simulink model "real_motor_awp"  (R2025b)
settings: Solver=VariableStepAuto  StartTime=0.0  StopTime=3  RelTol=1e-3
undefined symbols (not defined in the file): C, F, fc, G, K, K_awp, K_I, L, T, x_r
libraries: simulink x2
settings Model: Creator=noeliarosales  LastModifiedBy=noeliarosales

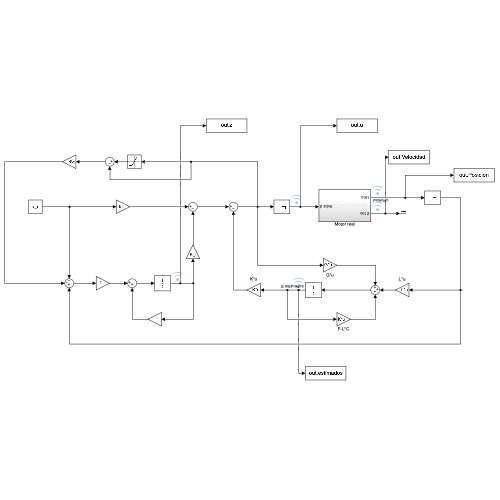
[thumbnail: Simulink's stored preview of the top-level diagram]
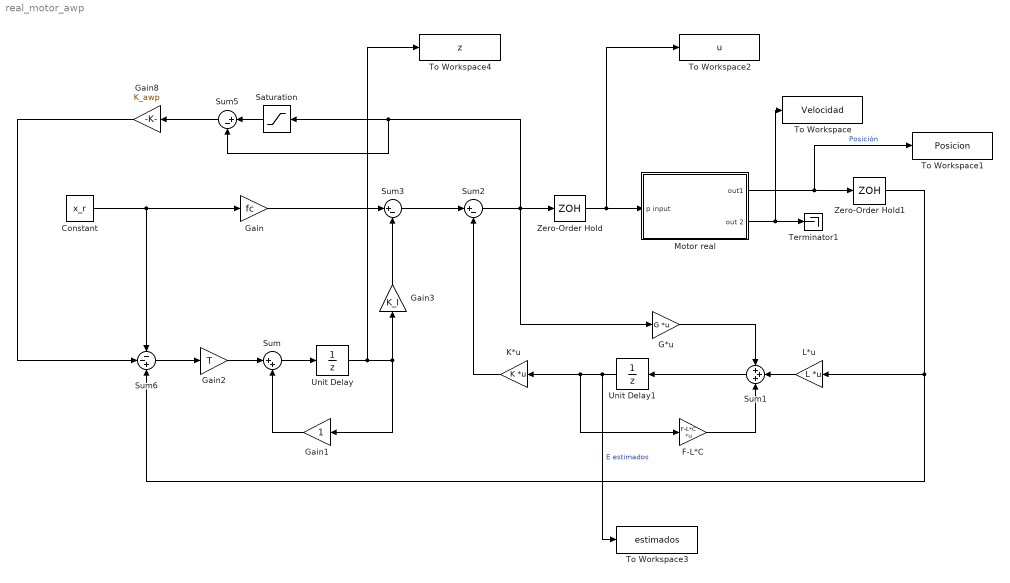
== system real_motor_awp ==
  Constant : Constant  Value=x_r
  F-L*C : Gain  Gain=F-L*C  Multiplication=Matrix(K*u)
  G*u : Gain  Gain=G  Multiplication=Matrix(K*u)
  Gain : Gain  Gain=fc
  Gain1 : Gain
  Gain2 : Gain  Gain=T
  Gain3 : Gain  Gain=K_I
  Gain8 : Gain  Gain=K_awp
  K*u : Gain  Gain=K  Multiplication=Matrix(K*u)
  L*u : Gain  Gain=L  Multiplication=Matrix(K*u)
  Motor real : Subsystem
  Saturation : Saturate  UpperLimit=100/12
  Sum : Sum  Inputs=|++
  Sum1 : Sum  Inputs=+++
  Sum2 : Sum  Inputs=|+-
  Sum3 : Sum  Inputs=|+-
  Sum5 : Sum  Inputs=|+-
  Sum6 : Sum  Inputs=--+
  Terminator1 : Terminator
  To Workspace : ToWorkspace  VariableName=Velocidad  SaveFormat=Timeseries  SampleTime=-1
  To Workspace1 : ToWorkspace  VariableName=Posicion  SaveFormat=Timeseries  SampleTime=-1
  To Workspace2 : ToWorkspace  VariableName=u  SaveFormat=Timeseries  SampleTime=-1
  To Workspace3 : ToWorkspace  VariableName=estimados  SaveFormat=Timeseries  SampleTime=-1
  To Workspace4 : ToWorkspace  VariableName=z  SaveFormat=Timeseries  SampleTime=-1
  Unit Delay : UnitDelay  SampleTime=-1  HasFrameUpgradeWarning=on
  Unit Delay1 : UnitDelay  SampleTime=-1  HasFrameUpgradeWarning=on
  Zero-Order Hold : ZeroOrderHold  SampleTime=T
  Zero-Order Hold1 : ZeroOrderHold  SampleTime=T
  wires:
  Zero-Order Hold/1 -> To Workspace2/1, Motor real/1(p input)
  Zero-Order Hold1/1 -> Sum6/3, L*u/1
  L*u/1 -> Sum1/2
  G*u/1 -> Sum1/1
  Sum1/1 -> Unit Delay1/1
  Constant/1 -> Sum6/1, Gain/1
  Gain3/1 -> Sum3/2
  F-L*C/1 -> Sum1/3
  Sum6/1 -> Gain2/1
  Sum3/1 -> Sum2/1
  Unit Delay1/1 -> To Workspace3/1, K*u/1, F-L*C/1  "E estimados"
  Sum/1 -> Unit Delay/1
  Motor real/1(out1) -> To Workspace1/1, Zero-Order Hold1/1  "Posición"
  Gain/1 -> Sum3/1
  K*u/1 -> Sum2/2
  Gain1/1 -> Sum/2
  Sum2/1 -> Sum5/2, Saturation/1, G*u/1, Zero-Order Hold/1
  Motor real/2(out 2) -> To Workspace/1, Terminator1/1
  Gain2/1 -> Sum/1
  Unit Delay/1 -> To Workspace4/1, Gain3/1, Gain1/1
  Sum5/1 -> Gain8/1
  Saturation/1 -> Sum5/1
  Gain8/1 -> Sum6/2

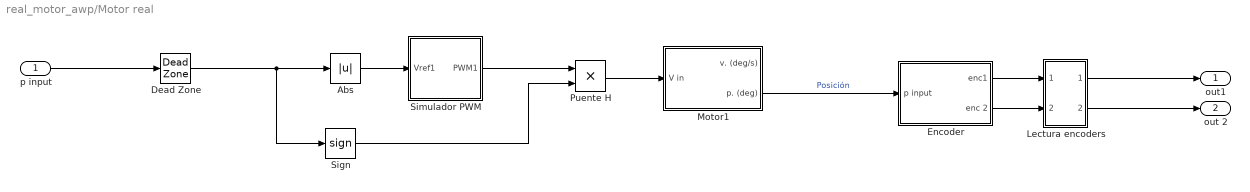
== system real_motor_awp/Motor real ==
  p input : Inport
  " Encoder" : Subsystem
  Abs : Abs  SaturateOnIntegerOverflow=off
  Dead Zone : DeadZone
  Lectura encoders : Subsystem
  Motor1 : Subsystem
  Puente H : Product
  Sign : Signum
  Simulador PWM : Subsystem
  out1 : Outport
  out 2 : Outport  Port=2
  wires:
  Lectura encoders/2(Encoder B) -> out 2/1
  Sign/1 -> Puente H/2
  Abs/1 -> Simulador PWM/1(Vref1)
  " Encoder"/1(enc1) -> Lectura encoders/1(enc1)
  " Encoder"/2(enc 2) -> Lectura encoders/2(enc 2)
  Puente H/1 -> Motor1/1(V in)
  Dead Zone/1 -> Sign/1, Abs/1
  Lectura encoders/1(Encoder A) -> out1/1
  Motor1/2(p. (deg)) -> " Encoder"/1(p input)  "Posición"
  Simulador PWM/1(PWM1) -> Puente H/1
  p input/1 -> Dead Zone/1

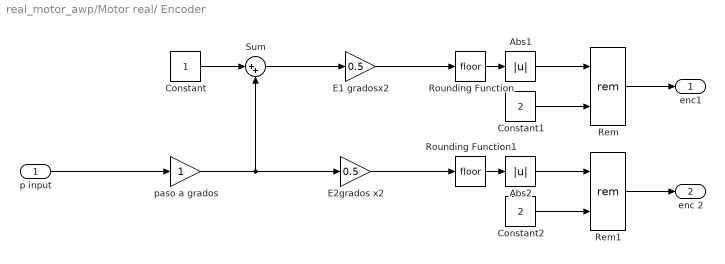
== system real_motor_awp/Motor real/ Encoder ==
  p input : Inport
  Abs1 : Abs  SaturateOnIntegerOverflow=off
  Abs2 : Abs  SaturateOnIntegerOverflow=off
  Constant : Constant
  Constant1 : Constant  Value=2
  Constant2 : Constant  Value=2
  E1 gradosx2 : Gain  Gain=0.5
  E2grados x2 : Gain  Gain=0.5
  Rem : Math  Operator=rem
  Rem1 : Math  Operator=rem
  Rounding Function : Rounding
  Rounding Function1 : Rounding
  Sum : Sum  Inputs=|++
  paso a grados : Gain
  enc1 : Outport
  enc 2 : Outport  Port=2
  wires:
  paso a grados/1 -> E2grados x2/1, Sum/2
  p input/1 -> paso a grados/1
  Sum/1 -> E1 gradosx2/1
  Constant/1 -> Sum/1
  E1 gradosx2/1 -> Rounding Function/1
  E2grados x2/1 -> Rounding Function1/1
  Rounding Function/1 -> Abs1/1
  Abs1/1 -> Rem/1
  Constant1/1 -> Rem/2
  Rounding Function1/1 -> Abs2/1
  Abs2/1 -> Rem1/1
  Constant2/1 -> Rem1/2
  Rem1/1 -> enc 2/1
  Rem/1 -> enc1/1

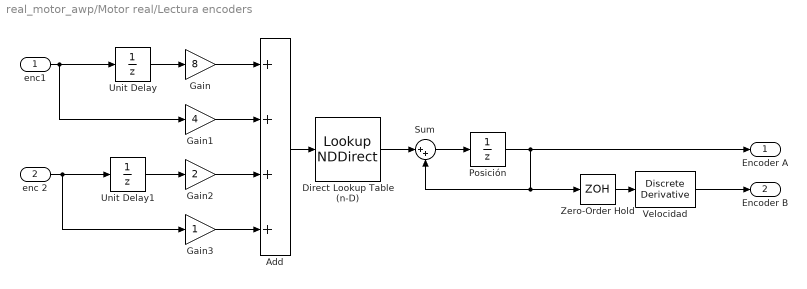
== system real_motor_awp/Motor real/Lectura encoders ==
  enc1 : Inport
  enc 2 : Inport  Port=2
  Add : Sum  Inputs=++++  OutDataTypeStr=double
  Direct Lookup Table (n-D) : LookupNDDirect  NumberOfTableDimensions=1  Table=[0,-1,1,0,1,0,0,-1,-1,0,0,1,0,1,-1,0]
  Gain : Gain  Gain=8
  Gain1 : Gain  Gain=4
  Gain2 : Gain  Gain=2
  Gain3 : Gain
  Posición : UnitDelay  SampleTime=-1  HasFrameUpgradeWarning=on
  Sum : Sum  Inputs=|++
  Unit Delay : UnitDelay  SampleTime=-1  HasFrameUpgradeWarning=on
  Unit Delay1 : UnitDelay  SampleTime=-1  HasFrameUpgradeWarning=on
  Velocidad : simulink/Discrete/Discrete Derivative  gainval=1.0  ICPrevScaledInput=0.0  OutMin=[]  OutMax=[]  OutDataType=fixdt(1, 16)  OutScaling=2^-10  DoSatur=off
  Zero-Order Hold : ZeroOrderHold  SampleTime=0.0001
  Encoder A : Outport
  Encoder B : Outport  Port=2
  wires:
  Add/1 -> Direct Lookup Table (n-D)/1
  Unit Delay/1 -> Gain/1
  enc 2/1 -> Gain3/1, Unit Delay1/1
  Sum/1 -> Posición/1
  Direct Lookup Table (n-D)/1 -> Sum/1
  Posición/1 -> Encoder A/1, Sum/2, Zero-Order Hold/1
  Zero-Order Hold/1 -> Velocidad/1
  Gain1/1 -> Add/2
  Gain3/1 -> Add/4
  Gain2/1 -> Add/3
  Unit Delay1/1 -> Gain2/1
  enc1/1 -> Unit Delay/1, Gain1/1
  Gain/1 -> Add/1
  Velocidad/1 -> Encoder B/1

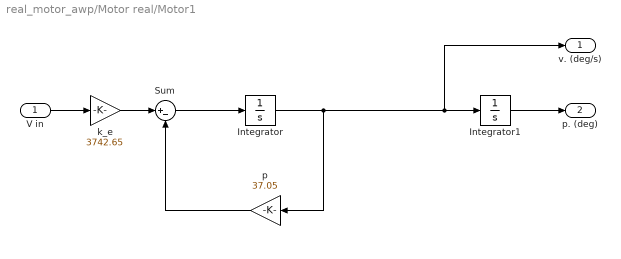
== system real_motor_awp/Motor real/Motor1 ==
  V in : Inport
  Integrator : Integrator
  Integrator1 : Integrator
  Sum : Sum  Inputs=|+-
  k_e : Gain  Gain=3742.65
  p : Gain  Gain=37.05
  v. (deg/s) : Outport
  p. (deg) : Outport  Port=2
  wires:
  p/1 -> Sum/2
  k_e/1 -> Sum/1
  Integrator/1 -> v. (deg/s)/1, Integrator1/1, p/1
  Integrator1/1 -> p. (deg)/1
  V in/1 -> k_e/1
  Sum/1 -> Integrator/1

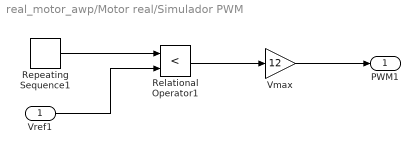
== system real_motor_awp/Motor real/Simulador PWM ==
  Vref1 : Inport
  Relational Operator1 : RelationalOperator  Operator=<  OutDataTypeStr=boolean  RndMeth=Simplest  InputSameDT=off
  Repeating Sequence1 : simulink/Sources/Repeating Sequence  rep_seq_t=linspace(0,0.001,100)  rep_seq_y=linspace(0,12,100)
  Vmax : Gain  Gain=12
  PWM1 : Outport
  wires:
  Relational Operator1/1 -> Vmax/1
  Vmax/1 -> PWM1/1
  Vref1/1 -> Relational Operator1/2
  Repeating Sequence1/1 -> Relational Operator1/1
